simulink model "supercond_cavity_CalPoly"  (Simulink 7.9)
settings: Solver=FixedStepDiscrete  StartTime=0.0  StopTime=Tfinal  FixedStep=Ts  RelTol=1e-3
values from neighbouring files (symbols this model uses):
  Ts = 1/fs    (= 2e-07)    [supercond_cavity_setup.m]
undefined symbols (not defined in the file or in its folder): prm
libraries: simulink x1
settings Model: Creator=claudio  LastModifiedBy=claudio

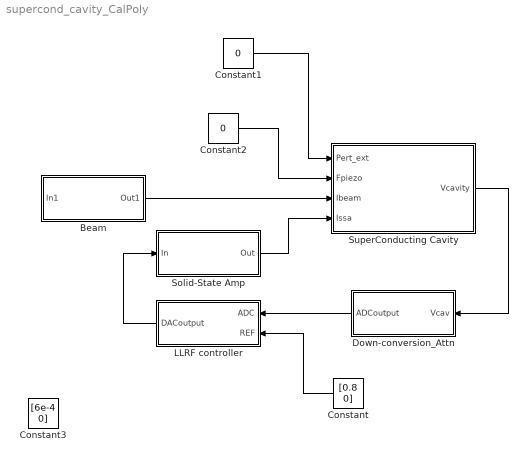
== system supercond_cavity_CalPoly ==
  Beam : Subsystem
  Constant : Constant  Value=[0.8 0]
  Constant1 : Constant  Value=0
  Constant2 : Constant  Value=0
  Constant3 : Constant  Value=[6e-4 0]
  Down-conversion_Attn : Subsystem
  LLRF controller : Subsystem
  Solid-State Amp : Subsystem
  SuperConducting Cavity : Subsystem
  wires:
  SuperConducting Cavity/1(Vcavity) -> Down-conversion_Attn/1(Vcav)
  Beam/1(Out1) -> SuperConducting Cavity/3(Ibeam)
  Down-conversion_Attn/1(ADCoutput) -> LLRF controller/1(ADC)
  Constant/1 -> LLRF controller/2(REF)
  Constant2/1 -> SuperConducting Cavity/2(Fpiezo)
  Constant1/1 -> SuperConducting Cavity/1(Pert_ext)
  LLRF controller/1(DACoutput) -> Solid-State Amp/1(In)
  Solid-State Amp/1(Out) -> SuperConducting Cavity/4(Issa)

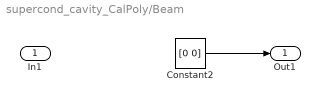
== system supercond_cavity_CalPoly/Beam ==
  In1 : Inport
  Constant2 : Constant  Value=[0 0]
  Out1 : Outport
  wires:
  Constant2/1 -> Out1/1

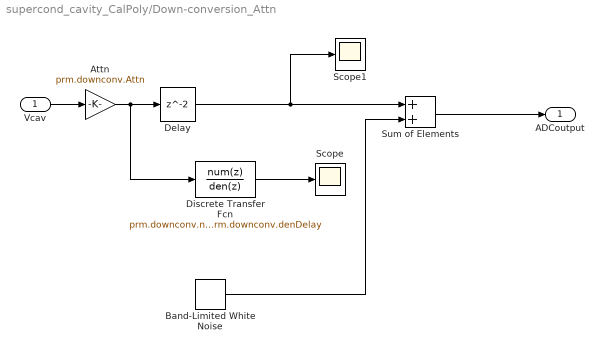
== system supercond_cavity_CalPoly/Down-conversion_Attn ==
  Vcav : Inport
  Attn : Gain  Gain=prm.downconv.Attn
  Band-Limited White Noise : simulink/Sources/Band-Limited White Noise  Cov=[0.0]  Ts=Ts  seed=[23341]
  Delay : Delay
  Discrete Transfer Fcn : DiscreteTransferFcn  Numerator=prm.downconv.numDelay  Denominator=prm.downconv.denDelay
  Scope : Scope
  Scope1 : Scope
      settings: SaveName=ScopeData6
  Sum of Elements : Sum
  ADCoutput : Outport
  wires:
  Vcav/1 -> Attn/1
  Attn/1 -> Delay/1, Discrete Transfer Fcn/1
  Sum of Elements/1 -> ADCoutput/1
  Band-Limited White Noise/1 -> Sum of Elements/2
  Delay/1 -> Sum of Elements/1, Scope1/1
  Discrete Transfer Fcn/1 -> Scope/1

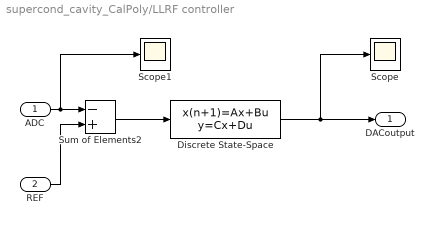
== system supercond_cavity_CalPoly/LLRF controller ==
  ADC : Inport
  REF : Inport  Port=2
  Discrete State-Space : DiscreteStateSpace  A=prm.LLRF.Api_D  B=prm.LLRF.Bpi_D  C=prm.LLRF.Cpi_D  D=prm.LLRF.Dpi_D  SampleTime=-1
  Scope : Scope
  Scope1 : Scope
      settings: SaveName=ScopeData5
  Sum of Elements2 : Sum  Inputs=-+
  DACoutput : Outport
  wires:
  Sum of Elements2/1 -> Discrete State-Space/1
  ADC/1 -> Sum of Elements2/1, Scope1/1
  REF/1 -> Sum of Elements2/2
  Discrete State-Space/1 -> DACoutput/1, Scope/1

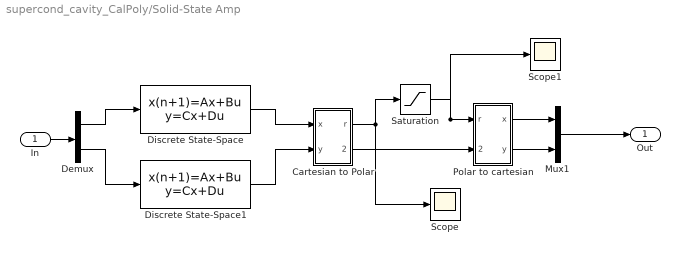
== system supercond_cavity_CalPoly/Solid-State Amp ==
  In : Inport
  Cartesian to Polar : Subsystem
      mask Type: [x,y]->[r,theta]
      mask Description:
      | Tranformation from cartesian to polar
      | coordinates.
      | r=sqrt(x^2+y^2), theta=atan(y/x)
      mask Help: Unmask this block for more help.
      mask Display: plot(0,0,100,100,[24,20,15,20,20],[85,95,85,95,20],[80,20,95,85,95,85],[70,20,20,15,20,24],[56,56,55,52,50,46],[20,26,31,35,38,42])
  Demux : Demux  Outputs=2
  Discrete State-Space : DiscreteStateSpace  A=prm.SSA.Assa  B=prm.SSA.Bssa  C=prm.SSA.Cssa  D=prm.SSA.Dssa  SampleTime=-1
  Discrete State-Space1 : DiscreteStateSpace  A=prm.SSA.Assa  B=prm.SSA.Bssa  C=prm.SSA.Cssa  D=prm.SSA.Dssa  SampleTime=-1
  Mux1 : Mux  Inputs=2
  Polar to cartesian : Subsystem
      mask Type: [r,theta]->[x,y]
      mask Description:
      | Tranformation from polar to cartesian
      | coordinates.
      | x=rcos(theta), y=rsin(theta)
      mask Help: Unmask this block for more help.
      mask Display: plot(0,0,100,100,[25,20,15,20,20],[85,95,85,95,20],[70,20,95,86,95,85],[60,20,20,15,20,25],[70,70],[45,54],[70,70],[30,40],[70,70],[20,25],[55,65],[60,60],[40,50],[60,60],[25,34],[60,60],[20,21],[60,60],[70,70,68],[57,60,60])
  Saturation : Saturate  UpperLimit=prm.SSA.Lmax  LowerLimit=prm.SSA.Lmin
  Scope : Scope
  Scope1 : Scope
      settings: SaveName=ScopeData2
  Out : Outport
  wires:
  Cartesian to Polar/1(r) -> Saturation/1, Scope/1
  Saturation/1 -> Polar to cartesian/1("r "), Scope1/1
  Cartesian to Polar/2(theta) -> Polar to cartesian/2("theta ")
  Mux1/1 -> Out/1
  Polar to cartesian/1(x) -> Mux1/1
  Polar to cartesian/2(y) -> Mux1/2
  In/1 -> Demux/1
  Demux/1 -> Discrete State-Space/1
  Discrete State-Space/1 -> Cartesian to Polar/1(x)
  Demux/2 -> Discrete State-Space1/1
  Discrete State-Space1/1 -> Cartesian to Polar/2(y)

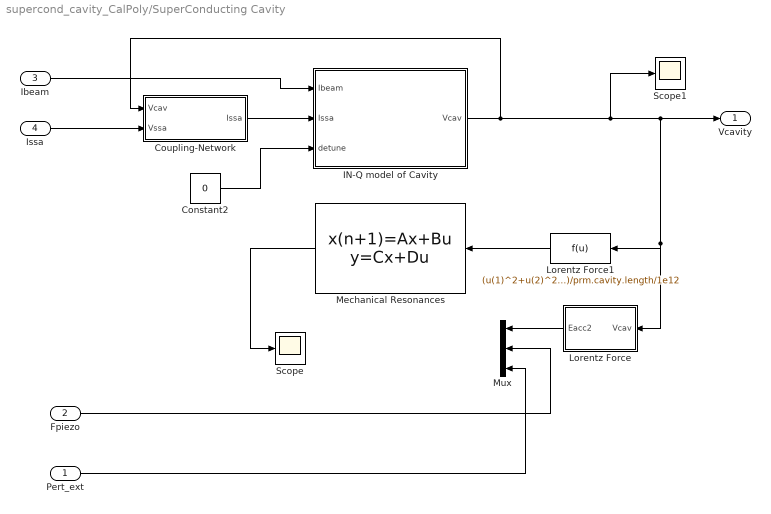
== system supercond_cavity_CalPoly/SuperConducting Cavity ==
  Pert_ext : Inport
  Fpiezo : Inport  Port=2
  Ibeam : Inport  Port=3
  Issa : Inport  Port=4
  Constant2 : Constant  Value=0
  Coupling-Network : Subsystem
  IN-Q model of Cavity : Subsystem
  Lorentz Force : Subsystem
  Lorentz Force1 : Fcn  Expr=(u(1)^2+u(2)^2)/prm.cavity.length/1e12
  Mechanical Resonances : DiscreteStateSpace  A=prm.mechanical.Amt  B=prm.mechanical.Bmt  C=prm.mechanical.Cmt  D=prm.mechanical.Dmt  X0=prm.mechanical.IC  SampleTime=-1
  Mux : Mux  Inputs=3
  Scope : Scope
      settings: SaveName=ScopeData3
  Scope1 : Scope
      settings: SaveName=ScopeData4
  Vcavity : Outport
  wires:
  IN-Q model of Cavity/1(Vcav) -> Vcavity/1, Lorentz Force/1(Vcav), Lorentz Force1/1, Scope1/1, Coupling-Network/1(Vcav)
  Ibeam/1 -> IN-Q model of Cavity/1(Ibeam)
  Fpiezo/1 -> Mux/2
  Pert_ext/1 -> Mux/3
  Lorentz Force/1(Eacc2) -> Mux/1
  Lorentz Force1/1 -> Mechanical Resonances/1
  Mechanical Resonances/1 -> Scope/1
  Coupling-Network/1(Issa) -> IN-Q model of Cavity/2(Issa)
  Issa/1 -> Coupling-Network/2(Vssa)
  Constant2/1 -> IN-Q model of Cavity/3(detune)

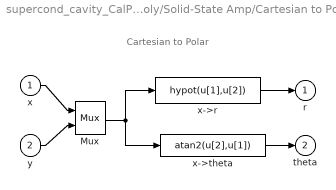
== system supercond_cavity_CalPoly/Solid-State Amp/Cartesian to Polar ==
  note: Cartesian to Polar
  x : Inport
  y : Inport  Port=2
  Mux : Mux  Inputs=2
  x->r : Fcn  Expr=hypot(u[1],u[2])
  x->theta : Fcn  Expr=atan2(u[2],u[1])
  r : Outport  InitialOutput=0
  theta : Outport  Port=2  InitialOutput=0
  wires:
  x->theta/1 -> theta/1
  y/1 -> Mux/2
  x/1 -> Mux/1
  x->r/1 -> r/1
  Mux/1 -> x->r/1, x->theta/1

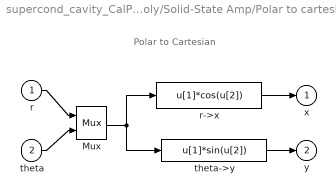
== system supercond_cavity_CalPoly/Solid-State Amp/Polar to cartesian ==
  note: Polar to Cartesian
  "r " : Inport
  "theta " : Inport  Port=2
  Mux : Mux  Inputs=2
  r->x : Fcn  Expr=u[1]*cos(u[2])
  theta->y : Fcn  Expr=u[1]*sin(u[2])
  x : Outport  InitialOutput=0
  y : Outport  Port=2  InitialOutput=0
  wires:
  Mux/1 -> r->x/1, theta->y/1
  r->x/1 -> x/1
  "r "/1 -> Mux/1
  "theta "/1 -> Mux/2
  theta->y/1 -> y/1

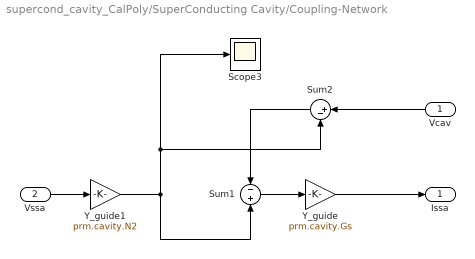
== system supercond_cavity_CalPoly/SuperConducting Cavity/Coupling-Network ==
  Vcav : Inport
  Vssa : Inport  Port=2
  Scope3 : Scope
      settings: YMin=-4.5e+06  YMax=750000  SaveName=ScopeData8
  Sum1 : Sum  Inputs=-+
  Sum2 : Sum  Inputs=|+-  SaturateOnIntegerOverflow=on
  Y_guide : Gain  Gain=prm.cavity.Gs
  Y_guide1 : Gain  Gain=prm.cavity.N2
  Issa : Outport
  wires:
  Sum1/1 -> Y_guide/1
  Sum2/1 -> Sum1/1
  Y_guide1/1 -> Sum1/2, Scope3/1, Sum2/2
  Y_guide/1 -> Issa/1
  Vssa/1 -> Y_guide1/1
  Vcav/1 -> Sum2/1

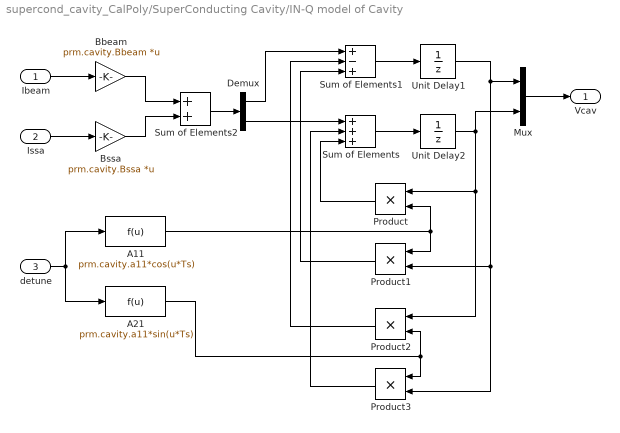
== system supercond_cavity_CalPoly/SuperConducting Cavity/IN-Q model of Cavity ==
  Ibeam : Inport
  Issa : Inport  Port=2
  detune : Inport  Port=3
  A11 : Fcn  Expr=prm.cavity.a11*cos(u*Ts)
  A21 : Fcn  Expr=prm.cavity.a11*sin(u*Ts)
  Bbeam : Gain  Gain=prm.cavity.Bbeam  Multiplication=Matrix(K*u)
  Bssa : Gain  Gain=prm.cavity.Bssa  Multiplication=Matrix(K*u)  SampleTime=Ts
  Demux : Demux  Outputs=2
  Mux : Mux  Inputs=2
  Product{,1..3} (4 alike) : Product  RndMeth=Zero
  Sum of Elements : Sum  Inputs=+++
  Sum of Elements1 : Sum  Inputs=+-+
  Sum of Elements2 : Sum
  Unit Delay1 : UnitDelay  SampleTime=-1
  Unit Delay2 : UnitDelay  SampleTime=-1
  Vcav : Outport
  wires:
  Mux/1 -> Vcav/1
  Issa/1 -> Bssa/1
  Ibeam/1 -> Bbeam/1
  Demux/1 -> Sum of Elements1/1
  Demux/2 -> Sum of Elements/1
  Sum of Elements2/1 -> Demux/1
  Bssa/1 -> Sum of Elements2/2
  Sum of Elements/1 -> Unit Delay2/1
  Sum of Elements1/1 -> Unit Delay1/1
  Unit Delay1/1 -> Mux/1, Product1/2, Product3/2
  Unit Delay2/1 -> Mux/2, Product/1, Product2/1
  detune/1 -> A11/1, A21/1
  Bbeam/1 -> Sum of Elements2/1
  A11/1 -> Product/2, Product1/1
  Product/1 -> Sum of Elements/3
  Product1/1 -> Sum of Elements1/3
  A21/1 -> Product3/1, Product2/2
  Product2/1 -> Sum of Elements1/2
  Product3/1 -> Sum of Elements/2

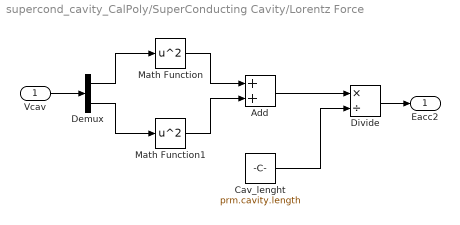
== system supercond_cavity_CalPoly/SuperConducting Cavity/Lorentz Force ==
  Vcav : Inport
  Add : Sum
  Cav_lenght : Constant  Value=prm.cavity.length
  Demux : Demux  Outputs=2
  Divide : Product  Inputs=*/
  Math Function : Math  Operator=square  SaturateOnIntegerOverflow=on
  Math Function1 : Math  Operator=square  SaturateOnIntegerOverflow=on
  Eacc2 : Outport
  wires:
  Vcav/1 -> Demux/1
  Divide/1 -> Eacc2/1
  Cav_lenght/1 -> Divide/2
  Add/1 -> Divide/1
  Math Function/1 -> Add/1
  Math Function1/1 -> Add/2
  Demux/1 -> Math Function/1
  Demux/2 -> Math Function1/1
